simulink subsystem "Sensor_Model"  (R2020a)
settings: Solver=VariableStepAuto  StartTime=0.0  StopTime=10.0  RelTol=1e-3
values from neighbouring files (symbols this model uses):
  xLp = [(xL(1) - padamount*gridsize):gridsize:xL(1)-gridsize, xL, xL(end)+gridsize:gridsize:xL(end)+padamount*gridsize]    [define_constants.m]
  yLp = [(yL(1) - padamount*gridsize):gridsize:yL(1)-gridsize, yL, yL(end)+gridsize:gridsize:yL(end)+padamount*gridsize]    [define_constants.m]
  Z = zeros(dims)    [define_constants.m]
undefined symbols (not defined in the file or in its folder): sunlightPattern
libraries: simulink x2
settings Model: Creator=alex  LastModifiedBy=matthewterblanche

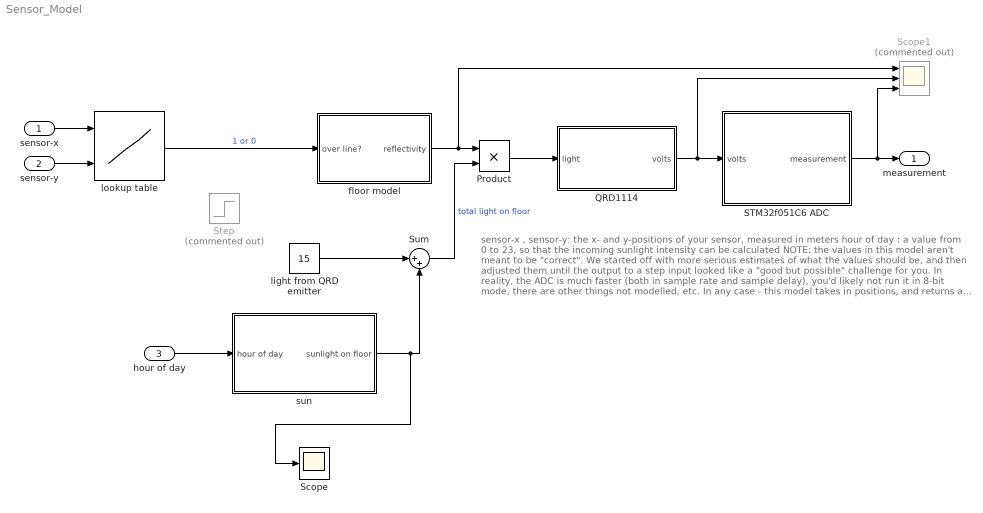
== system Sensor_Model ==
  note: sensor-x , sensor-y: the x- and y-positions of your sensor, measured in meters
      |
      | hour of day : a value from 0 to 23, so that the incoming sunlight intensity can be calculated
      |
      | NOTE: the values in this model aren't meant to be "correct". We started off with more serious estimates of what the values should be, and then adjusted them until the output to a step input looked like a "good but possible" challenge for you. In reality, the ADC is much faster (both in sample rate and sample delay), you'd likely not run it in 8-bit mode, there are other things not modelled, etc.
      |
      | In any case - this model takes in positions, and returns a sampled ADC measurement ranging from 0 to 1. You can disconnect the lookup table output, wire the step input into the floor model and uncomment the scope (see the image below) if you want to see what the intermediate signals look like. Don't forget to put things back afterwards, though!
  sensor-x : Inport
  sensor-y : Inport  Port=2
  hour of day : Inport  Port=3
  Product : Product
  QRD1114 : Subsystem
  STM32f051C6 ADC : Subsystem
  Scope : Scope
  Scope1 : Scope  Commented=on  NumInputPorts=3
  Step : Step  Commented=on  SampleTime=0
  Sum : Sum  Inputs=|++
  floor model : Subsystem
  light from QRD emitter : Constant  Value=15
  lookup table : Lookup_n-D  BreakpointsForDimension1=xLp  BreakpointsForDimension2=yLp  Table=transpose(Z)  InternalRulePriority=Speed  RndMeth=Simplest  InputSameDT=on
  sun : Subsystem
  measurement : Outport
  wires:
  sensor-x/1 -> lookup table/1
  sensor-y/1 -> lookup table/2
  lookup table/1 -> floor model/1(over line?)  "1 or 0"
  QRD1114/1(volts) -> STM32f051C6 ADC/1(volts), Scope1/2
  STM32f051C6 ADC/1(measurement) -> measurement/1, Scope1/3
  light from QRD emitter/1 -> Sum/1
  sun/1(sunlight on floor) -> Sum/2, Scope/1
  floor model/1(reflectivity) -> Product/1, Scope1/1
  Sum/1 -> Product/2  "total light on floor"
  Product/1 -> QRD1114/1(light)
  hour of day/1 -> sun/1(hour of day)

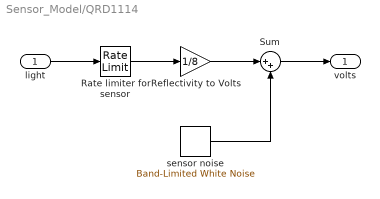
== system Sensor_Model/QRD1114 ==
  light : Inport
  Rate limiter for sensor : RateLimiter  RisingSlewLimit=1/(10^-6)  FallingSlewLimit=-1/(10^-6)  SampleTimeMode=inherited
  Reflectivity to Volts : Gain  Gain=1/8
  Sum : Sum  Inputs=|++
  sensor noise : simulink/Sources/Band-Limited White Noise  Cov=[0.000001]  Ts=0.001  seed=[23341]
  volts : Outport
  wires:
  sensor noise/1 -> Sum/2
  Sum/1 -> volts/1
  Reflectivity to Volts/1 -> Sum/1
  light/1 -> Rate limiter for sensor/1
  Rate limiter for sensor/1 -> Reflectivity to Volts/1

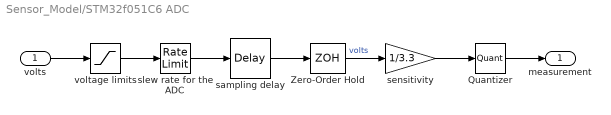
== system Sensor_Model/STM32f051C6 ADC ==
  volts : Inport
  Quantizer : Quantizer  QuantizationInterval=5/(2^8-1)
  Zero-Order Hold : ZeroOrderHold  SampleTime=0.005
  sampling delay : TransportDelay  DelayTime=0.005
  sensitivity : Gain  Gain=1/3.3
  slew rate for the ADC : RateLimiter  RisingSlewLimit=1000  FallingSlewLimit=-1000  SampleTimeMode=inherited
  voltage limits : Saturate  UpperLimit=3.3  LowerLimit=0
  measurement : Outport
  wires:
  Quantizer/1 -> measurement/1
  voltage limits/1 -> slew rate for the ADC/1
  sensitivity/1 -> Quantizer/1
  slew rate for the ADC/1 -> sampling delay/1
  volts/1 -> voltage limits/1
  sampling delay/1 -> Zero-Order Hold/1
  Zero-Order Hold/1 -> sensitivity/1  "volts"

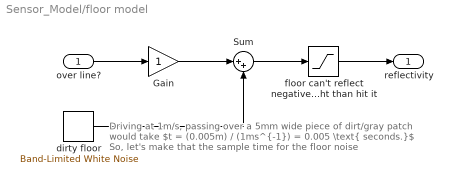
== system Sensor_Model/floor model ==
  note: Driving at 1m/s, passing over a 5mm wide piece of dirt/gray patch would take $t = (0.005m) / (1ms^{-1}) = 0.005 \text{ seconds.}$
      | So, let's make that the sample time for the floor noise
  over line? : Inport
  Gain : Gain
  Sum : Sum  Inputs=|++
  dirty floor : simulink/Sources/Band-Limited White Noise  Cov=[0.0001]  Ts=0.005  seed=[23341]
  floor can't reflect negative light or more light than hit it : Saturate  UpperLimit=1  LowerLimit=0
  reflectivity : Outport
  wires:
  floor can't reflect negative light or more light than hit it/1 -> reflectivity/1
  dirty floor/1 -> Sum/2
  Gain/1 -> Sum/1
  Sum/1 -> floor can't reflect negative light or more light than hit it/1
  over line?/1 -> Gain/1

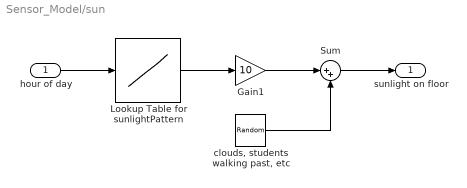
== system Sensor_Model/sun ==
  hour of day : Inport
  Gain1 : Gain  Gain=10
  Lookup Table for sunlightPattern : Lookup_n-D  NumberOfTableDimensions=1  BreakpointsForDimension1=0:23  Table=sunlightPattern  InternalRulePriority=Speed  RndMeth=Simplest  InputSameDT=on
  Sum : Sum  Inputs=|++
  "clouds, students walking past, etc" : UniformRandomNumber  Minimum=-2  Maximum=2  SampleTime=0.01
  sunlight on floor : Outport
  wires:
  "clouds, students walking past, etc"/1 -> Sum/2
  Gain1/1 -> Sum/1
  Sum/1 -> sunlight on floor/1
  hour of day/1 -> Lookup Table for sunlightPattern/1
  Lookup Table for sunlightPattern/1 -> Gain1/1
